simulink model "vezba_9ned"  (R2018a)
settings: Solver=VariableStepAuto  StartTime=0.0  StopTime=100  RelTol=1e-3
libraries: simulink x1
settings Model: Creator=Teodor  LastModifiedBy=Teodor

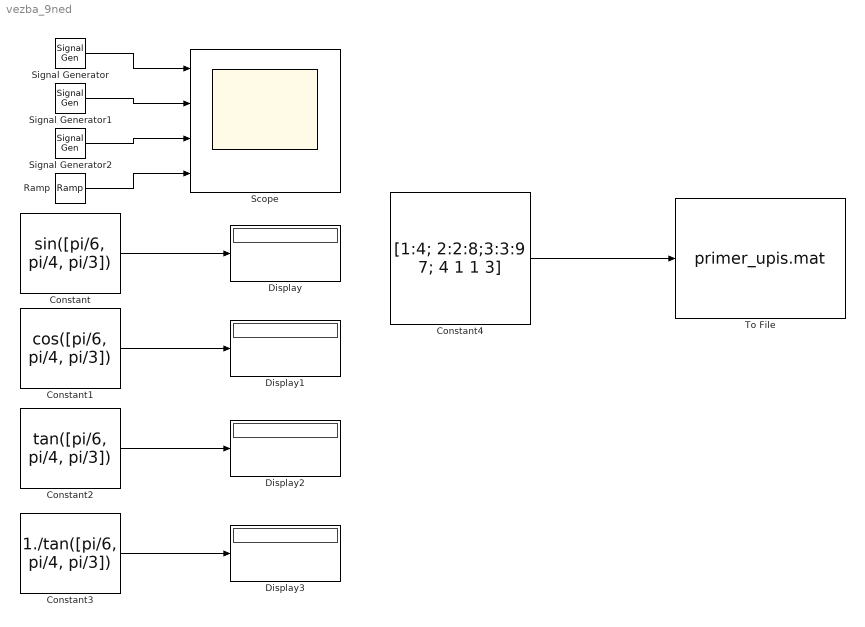
== system vezba_9ned ==
  Constant : Constant  Value=sin([pi/6, pi/4, pi/3])
  Constant1 : Constant  Value=cos([pi/6, pi/4, pi/3])
  Constant2 : Constant  Value=tan([pi/6, pi/4, pi/3])
  Constant3 : Constant  Value=1./tan([pi/6, pi/4, pi/3])
  Constant4 : Constant  Value=[1:4; 2:2:8;3:3:9 7; 4 1 1 3]
  Display{,1..3} (4 alike) : Display
  Ramp : simulink/Sources/Ramp  slope=5  start=20  InitialOutput=100
  Scope : Scope  NumInputPorts=4
  Signal Generator : SignalGenerator  Frequency=0.2  Units=rad/sec
  Signal Generator1 : SignalGenerator  WaveForm=square  Frequency=0.2  Units=rad/sec
  Signal Generator2 : SignalGenerator  WaveForm=sawtooth  Frequency=0.2  Units=rad/sec
  To File : ToFile  Filename=primer_upis.mat  MatrixName=matrica_A
  wires:
  Signal Generator/1 -> Scope/1
  Signal Generator1/1 -> Scope/2
  Signal Generator2/1 -> Scope/3
  Ramp/1 -> Scope/4
  Constant/1 -> Display/1
  Constant1/1 -> Display1/1
  Constant2/1 -> Display2/1
  Constant3/1 -> Display3/1
  Constant4/1 -> To File/1
